simulink model "PCC_NoGearOpt_Revision"  (R2020a)
settings: Solver=ode45  StartTime=0.0  StopTime=3000  RelTol=1e-3
PreLoadFcn:
  | initial
PostLoadFcn:
  | initial
InitFcn:
  | initial
model workspace (MAT data in the model file):
  Af : Simulink.Signal (value not decoded)
  CD : Simulink.Signal (value not decoded)
  Delta_t : Simulink.Signal (value not decoded)
  If : Simulink.Signal (value not decoded)
  Ig : Simulink.Signal (value not decoded)
  L00 : Simulink.Signal (value not decoded)
  L01 : Simulink.Signal (value not decoded)
  L02 : Simulink.Signal (value not decoded)
  L10 : Simulink.Signal (value not decoded)
  L11 : Simulink.Signal (value not decoded)
  L12 : Simulink.Signal (value not decoded)
  L20 : Simulink.Signal (value not decoded)
  L21 : Simulink.Signal (value not decoded)
  L22 : Simulink.Signal (value not decoded)
  M : Simulink.Signal (value not decoded)
  Np : Simulink.Signal (value not decoded)
  Tb_min : Simulink.Signal (value not decoded)
  Te_max : Simulink.Signal (value not decoded)
  Te_min : Simulink.Signal (value not decoded)
  eta : Simulink.Signal (value not decoded)
  f : Simulink.Signal (value not decoded)
  g : Simulink.Signal (value not decoded)
  kappa_1 : Simulink.Signal (value not decoded)
  kappa_2 : Simulink.Signal (value not decoded)
  rho : Simulink.Signal (value not decoded)
  rw : Simulink.Signal (value not decoded)
values from neighbouring files (symbols this model uses):
  EngMinTrq_Para_Value = -400    [initial.m]
  GearIni_Para_Value = 12    [initial.m]
  ParaMAP_RdSlopeOffsetAll = RdSlopeOffsetAll(5,1:2094)    [initial.m]
  ParaMAP_RdSlopeValueAll = RdSlopeValueAll(5,1:2094)    [initial.m]
  Rd_LeaderSpd = [19.4444444444 19.7511370506 20.5925623188 20.8767591057 20.2737444786 20.4902746731 20.4442142988 20.3221868298 20.2125924983 19.7727091401 19.6123069776 19.2200993307 ... (126 elements, 126x1)]    [RdLeaderSpdData.mat]
  Rd_Pos = [0:20:2500]    [LeaderSpd_Generate.m]    (also in RdLeaderSpdData.mat = [0 20 40 60 80 100 120 140 160 180 200 220 ... (126 elements)
undefined symbols (not defined in the file or in its folder): sigbuilder_block
libraries: simulink x4, Solver_SF x1
(part 2 of 2)

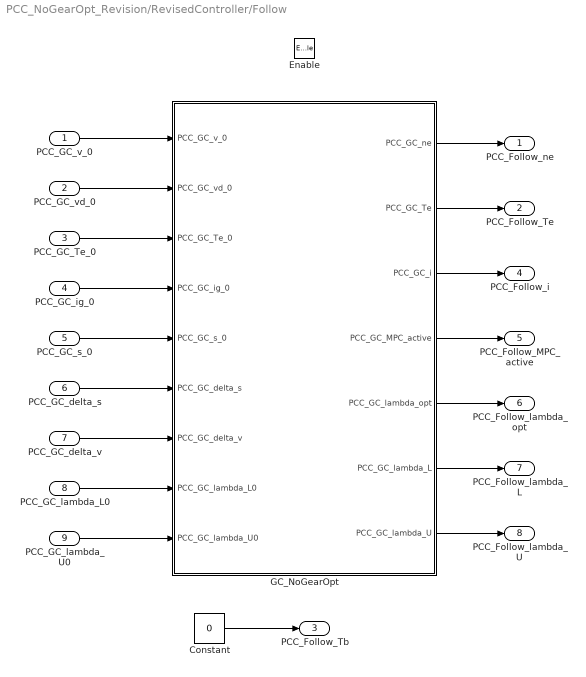
== system PCC_NoGearOpt_Revision/RevisedController/Follow ==
  PCC_GC_v_0 : Inport
  PCC_GC_vd_0 : Inport  Port=2
  PCC_GC_Te_0 : Inport  Port=3
  PCC_GC_ig_0 : Inport  Port=4
  PCC_GC_s_0 : Inport  Port=5
  PCC_GC_delta_s : Inport  Port=6
  PCC_GC_delta_v : Inport  Port=7
  PCC_GC_lambda_L0 : Inport  Port=8
  PCC_GC_lambda_U0 : Inport  Port=9
  Enable : EnablePort
  Constant : Constant  Value=0
  GC_NoGearOpt : MATLAB Function  TreatAsAtomicUnit=on
  PCC_Follow_ne : Outport
  PCC_Follow_Te : Outport  Port=2
  PCC_Follow_Tb : Outport  Port=3
  PCC_Follow_i : Outport  Port=4
  PCC_Follow_MPC_active : Outport  Port=5
  PCC_Follow_lambda_opt : Outport  Port=6
  PCC_Follow_lambda_L : Outport  Port=7
  PCC_Follow_lambda_U : Outport  Port=8
  wires:
  PCC_GC_Te_0/1 -> GC_NoGearOpt/3(PCC_GC_Te_0)
  GC_NoGearOpt/7(PCC_GC_lambda_U) -> PCC_Follow_lambda_U/1
  GC_NoGearOpt/6(PCC_GC_lambda_L) -> PCC_Follow_lambda_L/1
  PCC_GC_v_0/1 -> GC_NoGearOpt/1(PCC_GC_v_0)
  PCC_GC_s_0/1 -> GC_NoGearOpt/5(PCC_GC_s_0)
  PCC_GC_ig_0/1 -> GC_NoGearOpt/4(PCC_GC_ig_0)
  PCC_GC_delta_s/1 -> GC_NoGearOpt/6(PCC_GC_delta_s)
  PCC_GC_lambda_L0/1 -> GC_NoGearOpt/8(PCC_GC_lambda_L0)
  PCC_GC_lambda_U0/1 -> GC_NoGearOpt/9(PCC_GC_lambda_U0)
  PCC_GC_vd_0/1 -> GC_NoGearOpt/2(PCC_GC_vd_0)
  PCC_GC_delta_v/1 -> GC_NoGearOpt/7(PCC_GC_delta_v)
  GC_NoGearOpt/2(PCC_GC_Te) -> PCC_Follow_Te/1
  GC_NoGearOpt/1(PCC_GC_ne) -> PCC_Follow_ne/1
  GC_NoGearOpt/5(PCC_GC_lambda_opt) -> PCC_Follow_lambda_opt/1
  GC_NoGearOpt/3(PCC_GC_i) -> PCC_Follow_i/1
  GC_NoGearOpt/4(PCC_GC_MPC_active) -> PCC_Follow_MPC_active/1
  Constant/1 -> PCC_Follow_Tb/1

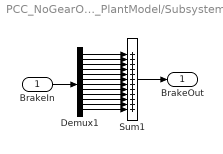
== system PCC_NoGearOpt_Revision/TruckSim_PlantModel/Subsystem ==
  BrakeIn : Inport
  Demux1 : Demux  Outputs=12
  Sum1 : Sum  Inputs=|++++++++++++
  BrakeOut : Outport  VectorParamsAs1DForOutWhenUnconnected=off
  wires:
  Demux1/5 -> Sum1/5
  Demux1/9 -> Sum1/9
  Demux1/6 -> Sum1/6
  Demux1/1 -> Sum1/1
  Demux1/7 -> Sum1/7
  Demux1/12 -> Sum1/12
  Demux1/10 -> Sum1/10
  Demux1/8 -> Sum1/8
  Demux1/3 -> Sum1/3
  Demux1/2 -> Sum1/2
  Demux1/11 -> Sum1/11
  Demux1/4 -> Sum1/4
  BrakeIn/1 -> Demux1/1
  Sum1/1 -> BrakeOut/1

== matlab function PCC_NoGearOpt_Revision/Subsystem1/MAPConstruction ==
  settings: updateMethod=DISCRETE
  data: PosIni output; Pos input; PosEnd output; RdSlpIni output; PosMry input; RdSlp input; count input; count output; SlpOffset_Para data_store_memory; SlpValue_Para data_store_memory
function [PosIni,PosEnd,RdSlpIni,count]= fcn(Pos,PosMry,RdSlp,count)

global SlpOffset_Para; 
global SlpValue_Para; 

if Pos>=fix(Pos/20)*20&&PosMry<fix(Pos/20)*20&&Pos>=SlpOffset_Para(end)
    PosTemp=zeros(200,1);
    SlpTemp=zeros(200,1);
    PosTemp(1:199)=SlpOffset_Para(2:end);
    PosTemp(200)=Pos;
    SlpTemp(1:199)=SlpValue_Para(2:end);
    SlpTemp(200)=RdSlp;
    SlpOffset_Para=PosTemp;
    SlpValue_Para=SlpTemp;
end

s_slp=SlpOffset_Para; %全局变量，当前位置距离初始位置的距离向量，坡度对应的距离
slp_r=SlpValue_Para; %全局变量，当前位置距离初始位置的坡度向量，坡度值
count_slp=max(size(SlpOffset_Para)); %当前位置距离初始位置的距离向量的数组长度
s_0=Pos-2000;
RdSlpIni=0;
i_slp_ini=1;
for counter_alpha=1:count_slp %插值得到当前位置对应坡度
    if(s_0>=s_slp(counter_alpha)&&s_0<s_slp(counter_alpha+1))
        RdSlpIni=slp_r(counter_alpha);
        i_slp_ini=counter_alpha;
        break
    end
end

PosIni = SlpOffset_Para(1);
PosEnd = SlpOffset_Para(200);

== matlab function PCC_NoGearOpt_Revision/RevisedController/Follow/GC_NoGearOpt ==
  settings: updateMethod=DISCRETE
  data: PCC_GC_ne output; PCC_GC_Te output; PCC_GC_i output; PCC_GC_MPC_active output; PCC_GC_lambda_opt output; PCC_GC_lambda_L output; PCC_GC_lambda_U output; PCC_GC_v_0 input; PCC_GC_vd_0 input; PCC_GC_Te_0 input; PCC_GC_ig_0 input; PCC_GC_s_0 input; PCC_GC_delta_s input; PCC_GC_delta_v input; SlpOffset_Para data_store_memory; SlpValue_Para data_store_memory; SpdLmtOffset_Para data_store_memory; SpdLmtValueU_Para data_store_memory; SpdLmtValueL_Para data_store_memory; PCC_GC_lambda_L0 input; PCC_GC_lambda_U0 input; Follow_Con_Para data_store_memory; Veh_Para data_store_memory; Trans_Para data_store_memory; FuelRate_Para data_store_memory; GearIni_Para data_store_memory; EngMaxSpd_Para data_store_memory; EngMaxTrq_Para data_store_memory; EngMinTrq_Para data_store_memory; EngMaxTrqFit_Para1 data_store_memory; EngMaxTrqFit_Para2 data_store_memory; EngMaxTrqFit_Para3 data_store_memory; EngMaxTrqFit_Para4 data_store_memory; ParaValue_Schedule data_store_memory
function [PCC_GC_ne,PCC_GC_Te,PCC_GC_i,PCC_GC_MPC_active,PCC_GC_lambda_opt,PCC_GC_lambda_L,PCC_GC_lambda_U] = Trucksim_Simulink_MPC_m_GenChe(PCC_GC_v_0,PCC_GC_vd_0,PCC_GC_Te_0,PCC_GC_ig_0,PCC_GC_s_0,PCC_GC_delta_s,PCC_GC_delta_v,PCC_GC_lambda_L0,PCC_GC_lambda_U0)
%% 全局变量-车辆固有参数&变速器传动比及初始档位赋值
% ---车辆固有参数---
global Veh_Para
rw=Veh_Para(8);
If=Veh_Para(9);
% ---变速器传动比---
global Trans_Para GearIni_Para
Ig=Trans_Para;
% ---档位赋值---
if PCC_GC_ig_0<Trans_Para(1)||PCC_GC_ig_0>length(Trans_Para)
    PCC_GC_ig_0=GearIni_Para; %初始化档位为14，避免刚仿真时档位为0
end
%% 全局变量-控制器参数，待标定
global Follow_Con_Para
kappa_2=Follow_Con_Para(2);%终端惩罚性指标权重系数
%% 道路信息赋值
% ---车速限速赋值---
global SpdLmtOffset_Para SpdLmtValueU_Para SpdLmtValueL_Para %引入全局变量，道路限速的距离向量，速度允许范围上边界，速度允许范围下边界
s_v=SpdLmtOffset_Para; %全局变量，道路限速的距离向量
v_max_r=SpdLmtValueU_Para; %全局变量，速度允许范围上边界
v_min_r=SpdLmtValueL_Para; %全局变量，速度允许范围下边界
count_v=max(size(SpdLmtOffset_Para)); %道路限速的距离向量的数组长度
% ---坡度赋值---
global SlpOffset_Para SlpValue_Para %引入全局变量，当前位置距离初始位置的距离向量，坡度对应的距离；当前位置距离初始位置的坡度向量，坡度值
s_alpha=SlpOffset_Para; %全局变量，当前位置距离初始位置的距离向量，坡度对应的距离
alpha_r=SlpValue_Para; %全局变量，当前位置距离初始位置的坡度向量，坡度值
count_alpha=max(size(SlpOffset_Para)); %当前位置距离初始位置的距离向量的数组长度
% ---初始位置对应坡度---
alpha_ini=0;
i_alpha_ini=1;
for counter_alpha=1:count_alpha-1 %插值得到当前位置对应坡度
    if(PCC_GC_s_0>=s_alpha(counter_alpha)&&PCC_GC_s_0<s_alpha(counter_alpha+1))
        alpha_ini=alpha_r(counter_alpha)+(alpha_r(counter_alpha+1)-alpha_r(counter_alpha))*(PCC_GC_s_0-s_alpha(counter_alpha))/(s_alpha(counter_alpha+1)-s_alpha(counter_alpha));
        i_alpha_ini=counter_alpha;
        break
    end
end
%% MPC迭代求解相关参数赋初始值
Cn=Follow_Con_Para(6);%算法迭代最长次数
Np=Follow_Con_Para(5);%预测步长
tp=Follow_Con_Para(4);%预测时域
Delta_t=Follow_Con_Para(3);
v_1=PCC_GC_v_0; %下一时刻车速，初始值为当前时刻车速
Te_1=PCC_GC_Te_0; %MPC求解得到的第一步最优发动机力矩值，初始值赋值
Te_2=PCC_GC_Te_0; %MPC求解得到的第二步最优发动机力矩值，初始值赋值
%% 调度图
global ParaValue_Schedule
V_ref=ParaValue_Schedule(1,:);
Distance_follow=ParaValue_Schedule(2,:);
t_follow=Distance_follow./V_ref;%跟车时距
th=interp1(V_ref,t_follow,PCC_GC_v_0,'linear');
Distance=th*PCC_GC_v_0;
%% 预测前车车速
beta1=0.5;%前车速度预测参数
gama1=5;%前车速度预测参数
beta2=0.5;%前车速度预测参数
gama2=40;%前车速度预测参数
ap0=0;%前车加速度，这里暂且设为0
sp0=PCC_GC_delta_s;%当前时刻前车的位移，设定本车当前时刻的位移是0
vp0=PCC_GC_delta_v+PCC_GC_v_0;%当前时刻前车的速度
vp=ones(Np+1,1);%预测时域内前车速度
ap=ones(Np+1,1);%预测时域内前车加速度
sp=ones(Np+1,1);%预测时域内前车位移
vp(1)=vp0;
ap(1)=ap0;
sp(1)=sp0;
for j=1:Np
    if(ap0<=0)%预测模型
        ap(j)=ap0/(1+exp(-1*beta1*(vp(j)-gama1)));
    else
        ap(j)=ap0/(1+exp(beta2*(vp(j)-gama2)));
    end
    vp(j+1)=vp(j)+Delta_t*ap(j);
    if(vp(j+1)<=0)
        vp(j+1)=0;
    end
    sp(j+1)=sp(j)+Delta_t*vp(j);
end
%%*******************************************************************************************************************************************************%计算终端条件
Vmax1=(sp(Np+1)-PCC_GC_v_0*Delta_t-Distance)/tp;
Vn=min(PCC_GC_vd_0,Vmax1);
PCC_GC_vd_0 = Vn;
%% 二分法初始化
v_min=Veh_Para(10);
v_max=Veh_Para(11);
diff=Follow_Con_Para(7);
diff_Lmt=Follow_Con_Para(8);
PCC_GC_lambda_L=PCC_GC_lambda_L0-diff;
[lambda,v_i,~,~,~]=DichotomySolution_Follow(PCC_GC_lambda_L,PCC_GC_s_0,PCC_GC_vd_0,PCC_GC_v_0,PCC_GC_ig_0,i_alpha_ini,alpha_ini,count_alpha,alpha_r,s_alpha,count_v,s_v,v_min_r,v_max_r,v_min,v_max);
Term_L=lambda-2*kappa_2*(v_i-PCC_GC_vd_0);
PCC_GC_lambda_U=PCC_GC_lambda_U0+diff;
[lambda,v_i,~,~,~]=DichotomySolution_Follow(PCC_GC_lambda_U,PCC_GC_s_0,PCC_GC_vd_0,PCC_GC_v_0,PCC_GC_ig_0,i_alpha_ini,alpha_ini,count_alpha,alpha_r,s_alpha,count_v,s_v,v_min_r,v_max_r,v_min,v_max);
Term_U=lambda-2*kappa_2*(v_i-PCC_GC_vd_0);
if Term_L>0
    PCC_GC_lambda_L=PCC_GC_lambda_L0-diff_Lmt;
    [lambda,v_i,~,~,~]=DichotomySolution_Follow(PCC_GC_lambda_L,PCC_GC_s_0,PCC_GC_vd_0,PCC_GC_v_0,PCC_GC_ig_0,i_alpha_ini,alpha_ini,count_alpha,alpha_r,s_alpha,count_v,s_v,v_min_r,v_max_r,v_min,v_max);
    Term_L=lambda-2*kappa_2*(v_i-PCC_GC_vd_0);
end
if Term_U<0
    PCC_GC_lambda_U=PCC_GC_lambda_U0+diff_Lmt;
    [lambda,v_i,~,~,~]=DichotomySolution_Follow(PCC_GC_lambda_U,PCC_GC_s_0,PCC_GC_vd_0,PCC_GC_v_0,PCC_GC_ig_0,i_alpha_ini,alpha_ini,count_alpha,alpha_r,s_alpha,count_v,s_v,v_min_r,v_max_r,v_min,v_max);
    Term_U=lambda-2*kappa_2*(v_i-PCC_GC_vd_0);
end
lambda_L_ini=PCC_GC_lambda_L;lambda_U_ini=PCC_GC_lambda_U;
%% 二分法求解最优初始lambda
PCC_GC_lambda_opt=0;
lambda_f=Term_L;
PCC_GC_i=1;
if Term_L*Term_U<=0
    PCC_GC_MPC_active=1;
    for PCC_GC_i=1:Cn %迭代求解最优协态变量及最优控制变量
        lambda=PCC_GC_lambda_L+0.5*(PCC_GC_lambda_U-PCC_GC_lambda_L); %对二分区间进行二分，lambda取二分区间中间值     
        PCC_GC_lambda_opt=lambda;
        [lambda,v_i,v_1,Te_1,Te_2]=DichotomySolution_Follow(lambda,PCC_GC_s_0,PCC_GC_vd_0,PCC_GC_v_0,PCC_GC_ig_0,i_alpha_ini,alpha_ini,count_alpha,alpha_r,s_alpha,count_v,s_v,v_min_r,v_max_r,v_min,v_max);
        if(lambda_f*(lambda-2*kappa_2*(v_i-PCC_GC_vd_0))<=0) %判断跨越零点位置，若零点位于下边界与中点之间则将中点设置为上边界继续二分迭代
            PCC_GC_lambda_U=PCC_GC_lambda_L+0.5*(PCC_GC_lambda_U-PCC_GC_lambda_L);
        else
            PCC_GC_lambda_L=PCC_GC_lambda_L+0.5*(PCC_GC_lambda_U-PCC_GC_lambda_L); %判断跨越零点位置，若零点位于上边界与中点之间则将中点设置为下边界继续二分迭代
            lambda_f=lambda-2*kappa_2*(v_i-PCC_GC_vd_0);
        end
    end
    Te_u=(Te_1+Te_2)/2; %为保证发动机控制稳定性，输出力矩为第一步和第二步最优发动机力矩的平均值
else
    PCC_GC_MPC_active=0;%不符合二分法条件
    Te_u=PCC_GC_Te_0;%保持上一时刻结果
end
%% 输出结果
PCC_GC_ne=v_1*If*Ig(PCC_GC_ig_0)*30/pi/rw; %输出发动机转速
PCC_GC_Te=Te_u; %输出发动机力矩
if lambda_U_ini-lambda_L_ini>=10 %二分法初始边界过大
    PCC_GC_Te=PCC_GC_Te_0;%保持上一时刻结果
end

== matlab function PCC_NoGearOpt_Revision/RevisedController/Brake/MATLAB Function1 ==
  settings: updateMethod=DISCRETE
  data: Tb output; v_0 input; vf_rela_0 input; sf_rela_0 input; ParaValue_Schedule data_store_memory; ParaValue_Brake data_store_memory
function Tb  = Brake(v_0,vf_rela_0,sf_rela_0)
global ParaValue_Schedule ParaValue_Brake
V_ref=ParaValue_Schedule(1,:);
Distance_brake=ParaValue_Schedule(2,:);%制动启动后直至该时距才停止
V_rela=ParaValue_Schedule(5,:);
Distance_rela=ParaValue_Schedule(6,:);
%% 赋值处理
% Th=ParaValue_Brake(2);%车辆反应时间
% ah_max=ParaValue_Brake(3);%本车制动减速度
% ap_max=g;%前车制动减速度
Tb_min=-120000;
%Tb_1=0;%初始化
Distance_buffer=interp1(V_ref,Distance_brake,v_0,'linear');
d_rela=interp1(V_rela,Distance_rela,vf_rela_0);
%% 制动执行器
Kv=ParaValue_Brake(1);
Ks=ParaValue_Brake(5);
delta_s=sf_rela_0;
S_des=Distance_buffer-d_rela;
%%%%%%%核心制动%%%%%%%%%

Tb_1=Kv*vf_rela_0 + Ks*(delta_s-S_des);

if Tb_1>0
    Tb_1 = 0;
end
if Tb_1<Tb_min
    Tb_1=Tb_min;
end
Tb=Tb_1;

== matlab function PCC_NoGearOpt_Revision/RevisedController/Mode_change ==
  settings: updateMethod=DISCRETE
  data: Ego_Vel input; Mode_out output; LeaderRelaSpd input; LeaderRelaPos input; Leader_State input; Mode_in input; ParaValue_Schedule data_store_memory
function Mode_out = Mode_change(Ego_Vel,LeaderRelaSpd,LeaderRelaPos,Leader_State,Mode_in)
%Mode=1表示非跟车，Mode=2表示跟车，Mode=3表示滑行，Mode=4表示制动
global ParaValue_Schedule
V_ref=ParaValue_Schedule(1,:);
Distance_follow_exist=ParaValue_Schedule(2,:);
Distance_follow=ParaValue_Schedule(3,:);
Distance_safe=ParaValue_Schedule(4,:);
t_follow=Distance_follow./V_ref;%跟车时距
t_follow_exist=Distance_follow_exist./V_ref;%制动启动后直至该时距才停止
t_safe=Distance_safe./V_ref;%跟车与非跟车中间的过渡区
%% 相对距离相对车速标定
V_rela=ParaValue_Schedule(5,:);
Distance_rela=ParaValue_Schedule(6,:);
%%
Pos_diff=LeaderRelaPos;%实际的前车位置减本车位置
V_diff=LeaderRelaSpd;%前车车速减本车车速

d_follow=interp1(V_ref,Distance_follow,Ego_Vel,'linear');%跟车间距80
d_follow_exist=interp1(V_ref,Distance_follow_exist,Ego_Vel,'linear');%跟车与非跟车过渡中点
d_safe=interp1(V_ref,Distance_safe,Ego_Vel,'linear');%跟车安全距离
d_brake_exist=interp1(V_ref,Distance_follow_exist,Ego_Vel,'linear');

d_diff=interp1(V_rela,Distance_rela,V_diff,'linear');%曲线

%% PCC跟车模式

if Leader_State==1
    if V_diff>=0 %前车快
        if Pos_diff>d_follow-d_diff
            Mode_out=1;
        elseif Pos_diff<d_safe-d_diff
            Mode_out=3;
        else
            if Mode_in~=1
                Mode_out=2;
            else
                if Pos_diff>d_follow_exist-d_diff
                    Mode_out=1;
                else
                    Mode_out=2;
                end
            end
        end
    else%后车快
        if Pos_diff < d_safe-d_diff
            Mode_out=4;
        elseif Pos_diff > d_follow-d_diff
            Mode_out=1;
        else
            if Mode_in~=1
                Mode_out=2;
            else
                if Pos_diff > d_follow_exist-d_diff
                    Mode_out=1;
                else
                    Mode_out=2;
                end
            end
        end
    end
else
    Mode_out=1;
end
if Mode_in==4
    if Pos_diff < d_brake_exist - d_diff
        Mode_out=Mode_in;
    end

end
if Mode_in==3
    if Pos_diff<d_follow_exist-d_diff
        Mode_out=Mode_in;
    end
end
% if LeaderRelaSpd > 3/3.6
%         Mode_out=4;
% end 
% % 强制PCC非跟车
% Mode_out=1;

== matlab function PCC_NoGearOpt_Revision/RevisedController/Cruise/FGC_NoGearOpt ==
  settings: updateMethod=DISCRETE
  data: PCC_FGC_ne output; PCC_FGC_Te output; PCC_FGC_i output; PCC_FGC_MPC_active output; PCC_FGC_lambda_opt output; PCC_FGC_lambda_L output; PCC_FGC_lambda_U output; PCC_FGC_v_0 input; PCC_FGC_vd_0 input; PCC_FGC_Te_0 input; PCC_FGC_ig_0 input; PCC_FGC_s_0 input; SlpOffset_Para data_store_memory; SlpValue_Para data_store_memory; SpdLmtOffset_Para data_store_memory; SpdLmtValueU_Para data_store_memory; SpdLmtValueL_Para data_store_memory; PCC_FGC_lambda_L0 input; PCC_FGC_lambda_U0 input; Cruise_Con_Para data_store_memory; Veh_Para data_store_memory; Trans_Para data_store_memory; FuelRate_Para data_store_memory; GearIni_Para data_store_memory; EngMaxSpd_Para data_store_memory; EngMaxTrq_Para data_store_memory; EngMinTrq_Para data_store_memory; EngMaxTrqFit_Para1 data_store_memory; EngMaxTrqFit_Para2 data_store_memory; EngMaxTrqFit_Para3 data_store_memory; EngMaxTrqFit_Para4 data_store_memory
function [PCC_FGC_ne,PCC_FGC_Te,PCC_FGC_i,PCC_FGC_MPC_active,PCC_FGC_lambda_opt,PCC_FGC_lambda_L,PCC_FGC_lambda_U] = Trucksim_Simulink_MPC_m_FeiGenChe(PCC_FGC_v_0,PCC_FGC_vd_0,PCC_FGC_Te_0,PCC_FGC_ig_0,PCC_FGC_s_0,PCC_FGC_lambda_L0,PCC_FGC_lambda_U0)
%% 全局变量-车辆固有参数&变速器传动比及初始档位赋值
% ---车辆固有参数---
global Veh_Para
rw=Veh_Para(8);
If=Veh_Para(9);
% ---变速器传动比---
global Trans_Para GearIni_Para
Ig=Trans_Para;
% ---档位赋值---
if PCC_FGC_ig_0<Trans_Para(1)||PCC_FGC_ig_0>length(Trans_Para)
    PCC_FGC_ig_0=GearIni_Para; %初始化档位为14，避免刚仿真时档位为0
end
%% 全局变量-控制器参数，待标定
global Cruise_Con_Para
kappa_2=Cruise_Con_Para(2);%终端惩罚性指标权重系数
%% 道路信息赋值
% ---车速限速赋值---
global SpdLmtOffset_Para SpdLmtValueU_Para SpdLmtValueL_Para %引入全局变量，道路限速的距离向量，速度允许范围上边界，速度允许范围下边界
s_v=SpdLmtOffset_Para; %全局变量，道路限速的距离向量
v_max_r=SpdLmtValueU_Para; %全局变量，速度允许范围上边界
v_min_r=SpdLmtValueL_Para; %全局变量，速度允许范围下边界
count_v=max(size(SpdLmtOffset_Para)); %道路限速的距离向量的数组长度
% ---坡度赋值---
global SlpOffset_Para SlpValue_Para %引入全局变量，当前位置距离初始位置的距离向量，坡度对应的距离；当前位置距离初始位置的坡度向量，坡度值
s_alpha=SlpOffset_Para; %全局变量，当前位置距离初始位置的距离向量，坡度对应的距离
alpha_r=SlpValue_Para; %全局变量，当前位置距离初始位置的坡度向量，坡度值
count_alpha=max(size(SlpOffset_Para)); %当前位置距离初始位置的距离向量的数组长度
% ---初始位置对应坡度---
alpha_ini=0;
i_alpha_ini=1;
for counter_alpha=1:count_alpha-1 %插值得到当前位置对应坡度
    if(PCC_FGC_s_0>=s_alpha(counter_alpha)&&PCC_FGC_s_0<s_alpha(counter_alpha+1))
        alpha_ini=alpha_r(counter_alpha)+(alpha_r(counter_alpha+1)-alpha_r(counter_alpha))*(PCC_FGC_s_0-s_alpha(counter_alpha))/(s_alpha(counter_alpha+1)-s_alpha(counter_alpha));
        i_alpha_ini=counter_alpha;
        break
    end
end
%% MPC迭代求解相关参数赋初始值
Cn=Cruise_Con_Para(6);%算法迭代最长次数
v_1=PCC_FGC_v_0; %下一时刻车速，初始值为当前时刻车速
Te_1=PCC_FGC_Te_0; %MPC求解得到的第一步最优发动机力矩值，初始值赋值
Te_2=PCC_FGC_Te_0; %MPC求解得到的第二步最优发动机力矩值，初始值赋值
%% 二分法初始化
v_min=Veh_Para(10);
v_max=Veh_Para(11);
diff=Cruise_Con_Para(7);
diff_Lmt=Cruise_Con_Para(8);
PCC_FGC_lambda_L=PCC_FGC_lambda_L0-diff;
[lambda,v_i,~,~,~]=DichotomySolution_Cruise(PCC_FGC_lambda_L,PCC_FGC_s_0,PCC_FGC_vd_0,PCC_FGC_v_0,PCC_FGC_ig_0,i_alpha_ini,alpha_ini,count_alpha,alpha_r,s_alpha,count_v,s_v,v_min_r,v_max_r,v_min,v_max);
Term_L=lambda-2*kappa_2*(v_i-PCC_FGC_vd_0);
PCC_FGC_lambda_U=PCC_FGC_lambda_U0+diff;
[lambda,v_i,~,~,~]=DichotomySolution_Cruise(PCC_FGC_lambda_U,PCC_FGC_s_0,PCC_FGC_vd_0,PCC_FGC_v_0,PCC_FGC_ig_0,i_alpha_ini,alpha_ini,count_alpha,alpha_r,s_alpha,count_v,s_v,v_min_r,v_max_r,v_min,v_max);
Term_U=lambda-2*kappa_2*(v_i-PCC_FGC_vd_0);
if Term_L>0
    PCC_FGC_lambda_L=PCC_FGC_lambda_L0-diff_Lmt;
    [lambda,v_i,~,~,~]=DichotomySolution_Cruise(PCC_FGC_lambda_L,PCC_FGC_s_0,PCC_FGC_vd_0,PCC_FGC_v_0,PCC_FGC_ig_0,i_alpha_ini,alpha_ini,count_alpha,alpha_r,s_alpha,count_v,s_v,v_min_r,v_max_r,v_min,v_max);
    Term_L=lambda-2*kappa_2*(v_i-PCC_FGC_vd_0);
end
if Term_U<0
    PCC_FGC_lambda_U=PCC_FGC_lambda_U0+diff_Lmt;
    [lambda,v_i,~,~,~]=DichotomySolution_Cruise(PCC_FGC_lambda_U,PCC_FGC_s_0,PCC_FGC_vd_0,PCC_FGC_v_0,PCC_FGC_ig_0,i_alpha_ini,alpha_ini,count_alpha,alpha_r,s_alpha,count_v,s_v,v_min_r,v_max_r,v_min,v_max);
    Term_U=lambda-2*kappa_2*(v_i-PCC_FGC_vd_0);
end
lambda_L_ini=PCC_FGC_lambda_L;lambda_U_ini=PCC_FGC_lambda_U;
%% 二分法求解最优初始lambda
PCC_FGC_lambda_opt=0;
lambda_f=Term_L;
PCC_FGC_i=1;
if Term_L*Term_U<=0
    PCC_FGC_MPC_active=1;
    for PCC_FGC_i=1:Cn %迭代求解最优协态变量及最优控制变量
        lambda=PCC_FGC_lambda_L+0.5*(PCC_FGC_lambda_U-PCC_FGC_lambda_L); %对二分区间进行二分，lambda取二分区间中间值     
        PCC_FGC_lambda_opt=lambda;
        [lambda,v_i,v_1,Te_1,Te_2]=DichotomySolution_Cruise(lambda,PCC_FGC_s_0,PCC_FGC_vd_0,PCC_FGC_v_0,PCC_FGC_ig_0,i_alpha_ini,alpha_ini,count_alpha,alpha_r,s_alpha,count_v,s_v,v_min_r,v_max_r,v_min,v_max);
        if(lambda_f*(lambda-2*kappa_2*(v_i-PCC_FGC_vd_0))<=0) %判断跨越零点位置，若零点位于下边界与中点之间则将中点设置为上边界继续二分迭代
            PCC_FGC_lambda_U=PCC_FGC_lambda_L+0.5*(PCC_FGC_lambda_U-PCC_FGC_lambda_L);
        else
            PCC_FGC_lambda_L=PCC_FGC_lambda_L+0.5*(PCC_FGC_lambda_U-PCC_FGC_lambda_L); %判断跨越零点位置，若零点位于上边界与中点之间则将中点设置为下边界继续二分迭代
            lambda_f=lambda-2*kappa_2*(v_i-PCC_FGC_vd_0);
        end
    end
    Te_u=(Te_1+Te_2)/2; %为保证发动机控制稳定性，输出力矩为第一步和第二步最优发动机力矩的平均值
else
    PCC_FGC_MPC_active=0;%不符合二分法条件
    Te_u=PCC_FGC_Te_0;%保持上一时刻结果
end
%% 输出结果
PCC_FGC_ne=v_1*If*Ig(PCC_FGC_ig_0)*30/pi/rw; %输出发动机转速
PCC_FGC_Te=Te_u; %输出发动机力矩
if lambda_U_ini-lambda_L_ini>=10 %二分法初始边界过大
    PCC_FGC_Te=PCC_FGC_Te_0;%保持上一时刻结果
end

== matlab function PCC_NoGearOpt_Revision/TruckSim_PlantModel/MATLAB Function1 ==
  data: Te input; Ft output; ig input; Ig data_store_memory; eta data_store_memory; rw data_store_memory; If data_store_memory; Veh_Para data_store_memory; Trans_Para data_store_memory; GearIni_Para data_store_memory
function Ft = fcn(Te,ig)
global Veh_Para Trans_Para GearIni_Para
eta=Veh_Para(7);
rw=Veh_Para(8);
If=Veh_Para(9);
if ig==0
    ig=GearIni_Para;
end
% Ft=0;
Ft=Te*Trans_Para(ig)*If*eta/rw;
% if Te>=0
%     Ft=Te*Ig(ig)*If*eta/rw;
% else
%     Ft=Te*Ig(ig)*If/eta/rw;
% end
